simulink model "simulink2"  (R2015a)
settings: Solver=ode45  StartTime=0.0  StopTime=10.0  RelTol=1e-3
settings Model: Creator=Bojana Vasic  LastModifiedBy=Bojana Vasic

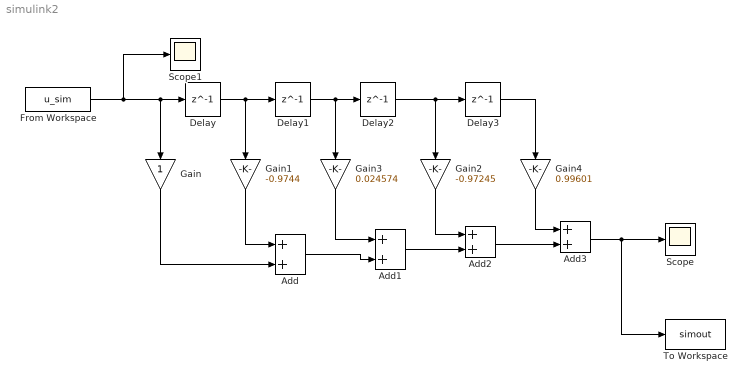
== system simulink2 ==
  Add{,1..3} (4 alike) : Sum
  Delay{,1..3} (4 alike) : Delay  DelayLength=1
  From Workspace : FromWorkspace  VariableName=u_sim  SampleTime=1
  Gain : Gain
  Gain1 : Gain  Gain=-0.9744
  Gain2 : Gain  Gain=-0.97245
  Gain3 : Gain  Gain=0.024574
  Gain4 : Gain  Gain=0.99601
  Scope : Scope
  Scope1 : Scope
  To Workspace : ToWorkspace  VariableName=simout  SaveFormat=Timeseries  SampleTime=-1
  wires:
  Gain/1 -> Add/2
  Gain1/1 -> Add/1
  Delay/1 -> Delay1/1, Gain1/1
  Gain3/1 -> Add1/1
  Add/1 -> Add1/2
  Delay1/1 -> Gain3/1, Delay2/1
  Delay2/1 -> Delay3/1, Gain2/1
  Gain2/1 -> Add2/1
  Add1/1 -> Add2/2
  Add2/1 -> Add3/2
  Delay3/1 -> Gain4/1
  Gain4/1 -> Add3/1
  Add3/1 -> Scope/1, To Workspace/1
  From Workspace/1 -> Scope1/1, Gain/1, Delay/1
